simulink model "quadrotor_ibvsTEST"  (R2016b)
settings: Solver=ode45  StartTime=0.0  StopTime=15  RelTol=1e-3  EnableMultiTasking=on
InitFcn:
  | mdl_aerialmanipulator
  | P =mkgrid(2, 0.1, transl(0,0,1));
  | Tcam = manipulator.fkine([0 3*pi/4 -pi/3 pi/4]);
  | 
  | 
  | q0 = [0 0 -pi/4 0]';
values from neighbouring files (symbols this model uses):
  manipulator = SerialLink([L1 L2 L3 L4], 'name', 'Arm')    [mdl_aerialmanipulator.m]
  ps = cam.project(Marker, 'Tcam', transl(CenterBias'+[0 0 TargetHeight])*trotx(-pi))    [mdl_aerialmanipulator.m]
undefined symbols (not defined in the file or in its folder): aerialmanipulator, r2t, rpy2tr, transl, trotx
libraries: roblocks x9
settings Model: Creator=zhonghang  LastModifiedBy=dell
settings DataIOCC: LimitDataPoints=on  SaveFormat=Array
settings OptimizationCC: LifeSpan=inf
settings DebuggingCC: SFUnexpectedBacktrackingDiag=warning  SFNoUnconditionalDefaultTransitionDiag=warning  SFExecutionAtInitializationDiag=none
settings HardwareCC: ProdBitPerPointer=32  ProdBitPerSizeT=32  ProdBitPerPtrDiffT=32  ProdLargestAtomicFloat=None  ProdIntDivRoundTo=Undefined  ProdEndianess=Unspecified  ProdWordSize=32  ProdHWDeviceType=32-bit Generic
settings ModelReferenceCC: PropagateSignalLabelsOutOfModel=off
settings GRTTargetCC: TargetLangStandard=C89/C90 (ANSI)  GeneratePreprocessorConditionals=Disable all
settings ConfigComp: CovMetricSettings=dw  CovHtmlReporting=on  CovSaveCumulativeToWorkspaceVar=on  CovSaveSingleToWorkspaceVar=on  CovExternalEMLEnable=off

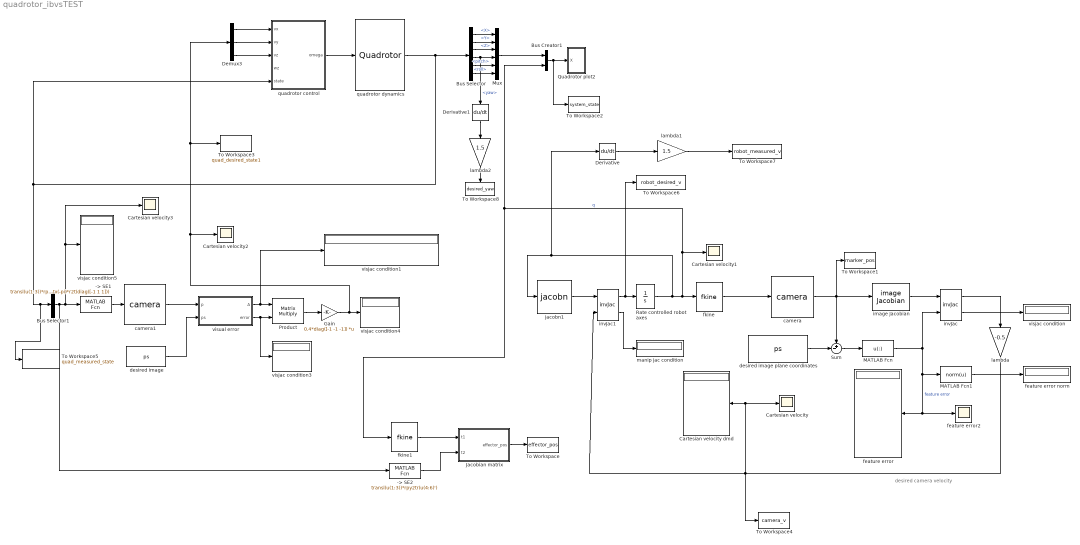
== system quadrotor_ibvsTEST ==
  note: desired camera velocity
  " Jacobian matrix" : MATLAB Function  TreatAsAtomicUnit=on
  -> SE1 : MATLABFcn  MATLABFcn=transl(u(1:3))*rpy2tr(u(4:6)')*trotx(-pi)*r2t(diag([-1 1 1]))  OutputDimensions=[4 4]  Output1D=off
  -> SE2 : MATLABFcn  MATLABFcn=transl(u(1:3))*rpy2tr(u(4:6)')  OutputDimensions=[4 4]  Output1D=off
  Bus Creator1 : BusCreator  Inputs=2
  Bus Selector : BusSelector  OutputSignals=X,Y,Z,yaw,pitch,roll
  Bus Selector1 : BusSelector  OutputSignals=X,Y,Z,roll,pitch,yaw  OutputAsBus=on
  Cartesian velocity{,1..3} (4 alike) : Scope
  Cartesian velocity dmd : Display
      settings: Format=bank
  Demux3 : Demux  Outputs=3
  Derivative : Derivative
  Derivative1 : Derivative
  Gain : Gain  Gain=0.4*diag([-1 -1 -1])  Multiplication=Matrix(K*u)
  MATLAB Fcn : MATLABFcn  MATLABFcn=u(:)  Output1D=off
  MATLAB Fcn1 : MATLABFcn  MATLABFcn=norm(u)
  Mux : Mux  Inputs=6
  Product : Product  Multiplication=Matrix(*)
  Quadrotor plot2 : Subsystem  AncestorBlock=roblocks/Robot Graphics/Quadrotor plot  mask{quad=aerialmanipulator, xydim=1, zdim=10}
      mask prompts: quad "Model"; xydim "xy-axes dimension"; zdim "z-axis dimension"
      mask help: Animate quadrotor.
      mask Help:
      | This block graphically displays a quadrotor (flying robot).
      | 
      | A new figure is created and A graphical model of a quadrotor is animated
      | to a pose specified by the state vector input to the block.
      | 
      | The state vector is [x y z roll pitch yaw] in world coordinates and the
      | angles are in radians.
      | 
      | Notes:
      | - The dimensions of the vehicle workspace are set by parameters
  Rate controlled robot axes : Integrator  InitialCondition=q0
  Sum : Sum  Inputs=+-|  SaturateOnIntegerOverflow=on  InputSameDT=on  OutDataTypeStr=Inherit: Same as first input
  To Workspace : ToWorkspace  VariableName=effector_pos  SaveFormat=Structure With Time  SampleTime=-1
  To Workspace1 : ToWorkspace  VariableName=marker_pos  SaveFormat=Structure With Time  SampleTime=-1
  To Workspace2 : ToWorkspace  VariableName=system_state  SaveFormat=Structure With Time  SampleTime=-1
  To Workspace3 : ToWorkspace  VariableName=quad_desired_state1  SaveFormat=Structure With Time  SampleTime=-1
  To Workspace4 : ToWorkspace  VariableName=camera_v  SaveFormat=Structure With Time  SampleTime=-1
  To Workspace5 : ToWorkspace  VariableName=quad_measured_state  SaveFormat=Structure With Time  SampleTime=-1
  To Workspace6 : ToWorkspace  VariableName=robot_desired_v  SaveFormat=Structure With Time  SampleTime=-1
  To Workspace7 : ToWorkspace  VariableName=robot_measured_v  SaveFormat=Structure With Time  SampleTime=-1
  To Workspace8 : ToWorkspace  VariableName=desired_yaw  SaveFormat=Structure With Time  SampleTime=-1
  camera : roblocks/Vision/camera  cam=cam  points=Marker
  camera1 : roblocks/Vision/camera  cam=cam  points=Marker
  desired image plane coordinates : Constant  Value=ps  VectorParams1D=off
  desired image : Constant  Value=ps  VectorParams1D=off
  feature error : Display
      settings: Format=bank
  feature error norm : Display
  feature error2 : Scope
  fkine : roblocks/Kinematics/fkine  robot=manipulator
  fkine1 : roblocks/Kinematics/fkine  robot=manipulator
  image Jacobian : roblocks/Vision/image Jacobian  cam=cam  z=2
  invJac : roblocks/Vision/invJac
  invJac1 : roblocks/Vision/invJac
  jacobn1 : roblocks/Kinematics/jacobn  robot=manipulator
  lambda : Gain  Gain=-0.5  SaturateOnIntegerOverflow=on  OutDataTypeStr=Inherit: Same as input  ParamDataTypeStr=Inherit: Same as input
  lambda1 : Gain  Gain=1.5  SaturateOnIntegerOverflow=on  OutDataTypeStr=Inherit: Same as input  ParamDataTypeStr=Inherit: Same as input
  lambda2 : Gain  Gain=1.5  SaturateOnIntegerOverflow=on  OutDataTypeStr=Inherit: Same as input  ParamDataTypeStr=Inherit: Same as input
  manip jac condition : Display
  quadrotor control : Subsystem
  quadrotor dynamics : roblocks/Dynamics/Quadrotor  quad=aerialmanipulator
      link override Dynamics: FunctionName=aerialmanipulator_dynamics
  visjac condition{,1,3..5} (5 alike) : Display
  visual error : MATLAB Function  TreatAsAtomicUnit=on
  wires:
  quadrotor control/1(omega) -> quadrotor dynamics/1
  Bus Creator1/1 -> To Workspace2/1, Quadrotor plot2/1(X)
  Bus Selector/1 -> Mux/1  "<X>"
  Bus Selector/2 -> Mux/2  "<Y>"
  Bus Selector/3 -> Mux/3  "<Z>"
  Bus Selector/4 -> Mux/4, Derivative1/1  "<yaw>"
  Bus Selector/5 -> Mux/5  "<pitch>"
  Bus Selector/6 -> Mux/6  "<roll>"
  Mux/1 -> Bus Creator1/1
  -> SE1/1 -> camera1/1
  quadrotor dynamics/1 -> Bus Selector/1, quadrotor control/5(state), To Workspace5/1, Bus Selector1/1
  camera1/1 -> visual error/1(p)
  desired image/1 -> visual error/2(ps)
  visual error/1(A) -> visjac condition1/1, Product/1
  Product/1 -> Gain/1
  Gain/1 -> To Workspace3/1, Demux3/1, Cartesian velocity2/1, visjac condition4/1
  visual error/2(error) -> visjac condition3/1, Product/2
  Bus Selector1/1 -> -> SE2/1, Cartesian velocity3/1, visjac condition5/1, -> SE1/1
  Rate controlled robot axes/1 -> fkine1/1, Bus Creator1/2, Cartesian velocity1/1, fkine/1, Derivative/1, jacobn1/1  "q"
  jacobn1/1 -> invJac1/1
  invJac1/1 -> To Workspace6/1, Rate controlled robot axes/1
  fkine/1 -> camera/1
  camera/1 -> To Workspace1/1, Sum/1, image Jacobian/1
  Sum/1 -> MATLAB Fcn/1
  desired image plane coordinates/1 -> Sum/2
  MATLAB Fcn/1 -> MATLAB Fcn1/1, feature error2/1, feature error/1, invJac/2  "feature error"
  invJac/2 -> visjac condition/1
  MATLAB Fcn1/1 -> feature error norm/1
  invJac/1 -> lambda/1
  image Jacobian/1 -> invJac/1
  lambda/1 -> To Workspace4/1, Cartesian velocity dmd/1, Cartesian velocity/1, invJac1/2
  invJac1/2 -> manip jac condition/1
  fkine1/1 -> " Jacobian matrix"/1(t1)
  -> SE2/1 -> " Jacobian matrix"/2(t2)
  " Jacobian matrix"/1(effector_pos) -> To Workspace/1
  Demux3/1 -> quadrotor control/1(vx)
  Demux3/2 -> quadrotor control/2(vy)
  Demux3/3 -> quadrotor control/3(vz)
  Derivative/1 -> lambda1/1
  lambda1/1 -> To Workspace7/1
  Derivative1/1 -> lambda2/1
  lambda2/1 -> To Workspace8/1

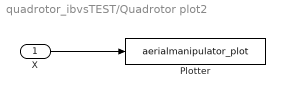
== system quadrotor_ibvsTEST/Quadrotor plot2 ==
  X : Inport
  Plotter : S-Function  FunctionName=aerialmanipulator_plot  Parameters=[xydim, zdim], 1, 1,aerialmanipulator  SFunctionDeploymentMode=off  EnableBusSupport=off
  wires:
  X/1 -> Plotter/1

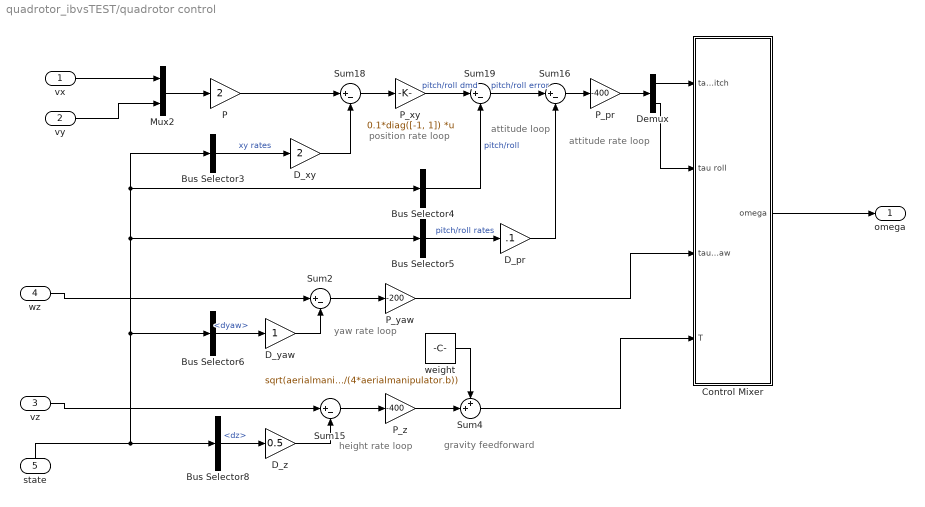
== system quadrotor_ibvsTEST/quadrotor control ==
  note: gravity feedforward
  note: attitude rate
      | loop
  note: attitude
      | loop
  note: position rate
      | loop
  note: yaw rate
      | loop
  note: height rate
      | loop
  vx : Inport
  vy : Inport  Port=2
  vz : Inport  Port=3
  wz : Inport  Port=4
  state : Inport  Port=5
  Bus Selector3 : BusSelector  OutputSignals=dx,dy  OutputAsBus=on
  Bus Selector4 : BusSelector  OutputSignals=pitch,roll  OutputAsBus=on
  Bus Selector5 : BusSelector  OutputSignals=dpitch,droll  OutputAsBus=on
  Bus Selector6 : BusSelector  OutputSignals=dyaw
  Bus Selector8 : BusSelector  OutputSignals=dz
  Control Mixer : Subsystem  AncestorBlock=roblocks/Dynamics/Control Mixer 4
      mask help: Quadrotor control mixer
      mask Help:
      | Determine rotor speeds based on desired torques and thrust.
      | 
      | <b>Inputs::</b>
      | 
      | tau pitch (1x1)  desired pitching torque [Nm]
      | tau roll (1x1)   desired rolling torque [Nm]
      | tau yaw (1x1)    desired yawing torque [Nm]
      | T (1x1)          desired thrust [N]
      | 
      | <b>Outputs::</b>
      | 
      | w1 (1x1) angular velocity of rotor 1 [rad]
      | w2 (1x1) angular velocity of rotor 2 [rad]
      | w3 (1x1) angular velocity of rotor 3 [rad]
      | w4 (1x1) angular velocity of rotor 4 [rad]
      | 
      | <b>Notes::</b>
      | 
      | - Assumes the rotor labelling convention of RVC Fig 4.16.
      | - The quadrotor is underactuated and has only 4 inputs.
  D_pr : Gain  Gain=.1
  D_xy : Gain  Gain=2
  D_yaw : Gain
  D_z : Gain  Gain=0.5
  Demux : Demux  Outputs=2
  Mux2 : Mux  Inputs=2
  P : Gain  Gain=2
  P_pr : Gain  Gain=-400
  P_xy : Gain  Gain=0.1*diag([-1, 1])  Multiplication=Matrix(K*u)
  P_yaw : Gain  Gain=-200
  P_z : Gain  Gain=-400
  Sum{2,15..16,18..19} (5 alike) : Sum  Inputs=|+-
  Sum4 : Sum  Inputs=++|
  weight : Constant  Value=sqrt(aerialmanipulator.M*aerialmanipulator.g/(4*aerialmanipulator.b))  SampleTime=0
  omega : Outport
  wires:
  state/1 -> Bus Selector8/1, Bus Selector5/1, Bus Selector4/1, Bus Selector3/1, Bus Selector6/1
  Mux2/1 -> P/1
  P/1 -> Sum18/1
  Sum18/1 -> P_xy/1
  wz/1 -> Sum2/1
  vz/1 -> Sum15/1
  Control Mixer/1(omega) -> omega/1
  Bus Selector3/1 -> D_xy/1  "xy rates"
  D_xy/1 -> Sum18/2
  P_xy/1 -> Sum19/1  "pitch/roll dmd"
  Bus Selector4/1 -> Sum19/2  "pitch/roll"
  Sum19/1 -> Sum16/1  "pitch/roll error"
  P_pr/1 -> Demux/1
  Bus Selector6/1 -> D_yaw/1  "<dyaw>"
  Bus Selector8/1 -> D_z/1  "<dz>"
  D_z/1 -> Sum15/2
  D_pr/1 -> Sum16/2
  Demux/2 -> Control Mixer/2(tau roll)
  Sum2/1 -> P_yaw/1
  P_yaw/1 -> Control Mixer/3(tau yaw)
  Demux/1 -> Control Mixer/1(tau pitch)
  Bus Selector5/1 -> D_pr/1  "pitch/roll rates"
  D_yaw/1 -> Sum2/2
  weight/1 -> Sum4/1
  Sum4/1 -> Control Mixer/4(T)
  vx/1 -> Mux2/1
  Sum16/1 -> P_pr/1
  vy/1 -> Mux2/2
  Sum15/1 -> P_z/1
  P_z/1 -> Sum4/2

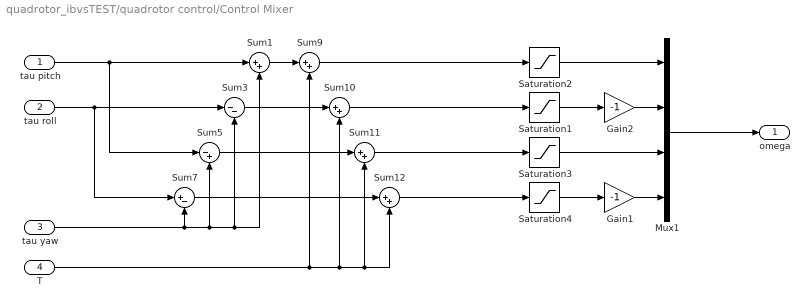
== system quadrotor_ibvsTEST/quadrotor control/Control Mixer ==
  tau pitch : Inport
  tau roll : Inport  Port=2
  tau yaw : Inport  Port=3
  T : Inport  Port=4
  Gain1 : Gain  Gain=-1
  Gain2 : Gain  Gain=-1
  Mux1 : Mux
  Saturation{1..4} (4 alike) : Saturate  UpperLimit=1000  LowerLimit=700
  Sum{1,9..12} (5 alike) : Sum  Inputs=|++  SaturateOnIntegerOverflow=on  InputSameDT=on  OutDataTypeStr=Inherit: Same as first input
  Sum3 : Sum  Inputs=|--  SaturateOnIntegerOverflow=on  InputSameDT=on  OutDataTypeStr=Inherit: Same as first input
  Sum5 : Sum  Inputs=|-+  SaturateOnIntegerOverflow=on  InputSameDT=on  OutDataTypeStr=Inherit: Same as first input
  Sum7 : Sum  Inputs=|+-  SaturateOnIntegerOverflow=on  InputSameDT=on  OutDataTypeStr=Inherit: Same as first input
  omega : Outport
  wires:
  Mux1/1 -> omega/1
  Gain2/1 -> Mux1/2
  tau yaw/1 -> Sum7/2, Sum5/2, Sum3/2, Sum1/2
  Saturation2/1 -> Mux1/1
  Saturation1/1 -> Gain2/1
  Saturation3/1 -> Mux1/3
  Saturation4/1 -> Gain1/1
  tau pitch/1 -> Sum1/1, Sum5/1
  Sum1/1 -> Sum9/1
  Sum3/1 -> Sum10/1
  Sum5/1 -> Sum11/1
  Sum7/1 -> Sum12/1
  Sum9/1 -> Saturation2/1
  Sum10/1 -> Saturation1/1
  Sum11/1 -> Saturation3/1
  Sum12/1 -> Saturation4/1
  T/1 -> Sum11/2, Sum12/2, Sum10/2, Sum9/2
  tau roll/1 -> Sum3/1, Sum7/1
  Gain1/1 -> Mux1/4

== matlab function quadrotor_ibvsTEST/ Jacobian matrix ==
  data: effector_pos output; t1 input; t2 input
function effector_pos  = JmainCal(t1, t2)
%#codegen

Base_T =[0.7071 0.7071 0 0; ...
    -0.7071 0.7071 0 0; ...
    0 0 -1.0000 0; ...
    0 0 0 1.0000];
s = t2*Base_T*t1;
effector_pos = s(1:3,4)';

== matlab function quadrotor_ibvsTEST/visual error ==
  data: A output; p input; error output; ps input
function [A, error] = visualerror(p, ps)
%% get the visual error message
% cal s and s*
[m,n] = size(p);
s = (1/500)*(p - repmat([640;400],[1 n]));
s = [s; ones(1,n)];
for i=1:n
    s(:,i) = s(:,i)./norm(s(:,i));
end
st = (1/500)*(ps - repmat([640;400],[1 n]));
st = [st; ones(1,n)];
for i=1:n
    st(:,i) = st(:,i)./norm(st(:,i));
end
% cal sum of s
h = sum(s,2);
ht = sum(st,2);
% delta h 
delta_h = h - ht;
%% modefied delta h
namda = 2;
ht_stat = ht./norm(ht);
% error = h - ht;
error = cross(ht_stat, h) + namda*ht_stat*(ht_stat'*delta_h);
%% A for use
sk_ht = [0 -ht_stat(3) ht_stat(2);...
    ht_stat(3) 0 -ht_stat(1);...
    -ht_stat(2) ht_stat(1) 0];
A = -sk_ht + namda*(ht_stat*ht_stat');
